simulink model "open_vs_closed_simulink_control101"  (R2024a)
settings: Solver=VariableStepAuto  StartTime=0.0  StopTime=endtime  RelTol=1e-3
undefined symbols (not defined in the file): den, Kden, Knum, num
settings Model: Creator=Anthony Rossiter  LastModifiedBy=Anthony Rossiter

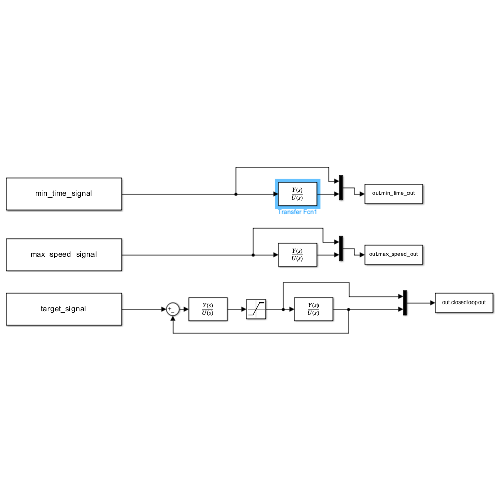
[thumbnail: Simulink's stored preview of the top-level diagram]
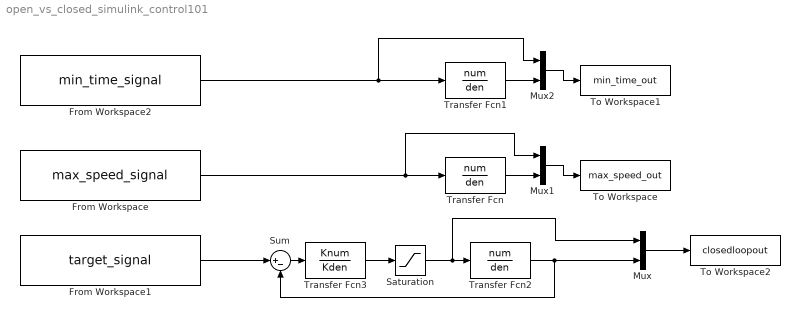
== system open_vs_closed_simulink_control101 ==
  From Workspace : FromWorkspace  VariableName=max_speed_signal
  From Workspace1 : FromWorkspace  VariableName=target_signal
  From Workspace2 : FromWorkspace  VariableName=min_time_signal
  Mux : Mux  Inputs=2
  Mux1 : Mux  Inputs=2
  Mux2 : Mux  Inputs=2
  Saturation : Saturate  UpperLimit=1  LowerLimit=-1
  Sum : Sum  Inputs=|+-
  To Workspace : ToWorkspace  VariableName=max_speed_out  SaveFormat=Timeseries  SampleTime=-1
  To Workspace1 : ToWorkspace  VariableName=min_time_out  SaveFormat=Timeseries  SampleTime=-1
  To Workspace2 : ToWorkspace  VariableName=closedloopout  SaveFormat=Timeseries  SampleTime=-1
  Transfer Fcn : TransferFcn  Numerator=num  Denominator=den
  Transfer Fcn1 : TransferFcn  Numerator=num  Denominator=den
  Transfer Fcn2 : TransferFcn  Numerator=num  Denominator=den
  Transfer Fcn3 : TransferFcn  Numerator=Knum  Denominator=Kden
  wires:
  From Workspace/1 -> Mux1/1, Transfer Fcn/1
  From Workspace1/1 -> Sum/1
  Transfer Fcn2/1 -> Mux/2, Sum/2
  Transfer Fcn3/1 -> Saturation/1
  Sum/1 -> Transfer Fcn3/1
  Saturation/1 -> Mux/1, Transfer Fcn2/1
  From Workspace2/1 -> Mux2/1, Transfer Fcn1/1
  Mux/1 -> To Workspace2/1
  Transfer Fcn1/1 -> Mux2/2
  Mux2/1 -> To Workspace1/1
  Transfer Fcn/1 -> Mux1/2
  Mux1/1 -> To Workspace/1
